simulink model "two_tank_simple"  (R2023b)
settings: Solver=ode45  StartTime=0.0  StopTime=199.9  RelTol=1e-3  EnableMultiTasking=on
values from neighbouring files (symbols this model uses):
  A1 = 0.0154    [INIT.m]
  A2 = 0.0154    [INIT.m]
  Cvb = 1.5938*1e-4    (= 0.00015938)    [INIT.m]
  Cvo = 1.59640*1e-4    (= 0.00015964)    [INIT.m]
  h1c = 0.5    [INIT.m]
  h1c_0 = 0    [INIT.m]
  h1max = 0.6    [INIT.m]
  h2c_0 = 0.03    [INIT.m]
  h2c_max = 0.11    [INIT.m]
  h2c_min = 0.09    [INIT.m]
  h2max = 0.6    [INIT.m]
  Ki = 5*1e-6    (= 5e-06)    [INIT.m]
  Kp = 1e-3    (= 0.001)    [INIT.m]
  Qf1 = 1e-4    (= 0.0001)    [INIT.m]    (also in extract_data.m = 5e-5*randn + 1e-4)
  Qf2 = 1e-4    (= 0.0001)    [INIT.m]    (also in extract_data.m = 5e-5*randn + 1e-4)
  Qpmax = 1e-2    (= 0.01)    [INIT.m]
  rate_noise_mQp = 1e-6    (= 1e-06)    [INIT.m]
  rate_noise_mUp = 1e-6    (= 1e-06)    [INIT.m]
  rate_noise_my1 = 1e-6    (= 1e-06)    [INIT.m]
  rate_noise_my2 = 1e-6    (= 1e-06)    [INIT.m]
  Te = 1    [INIT.m]
  yo = 0    [INIT.m]
(part 1 of 4)
settings Model: Creator=upcnet  LastModifiedBy=Plambeck
settings SolverCC: AlgebraicLoopSolver=TrustRegion
settings DataIOCC: LimitDataPoints=on  SaveFormat=Array  SignalLoggingSaveFormat=ModelDataLogs  ReturnWorkspaceOutputs=off  SignalLoggingName=sigsOut
settings OptimizationCC: BlockReduction=off  BooleanDataType=off  LifeSpan=inf
settings DebuggingCC: SaveWithParameterizedLinksMsg=none  UnderspecifiedInitializationDetection=Classic  MergeDetectMultiDrivingBlocksExec=none  SignalResolutionControl=TryResolveAllWithWarning  MultiTaskDSMMsg=warning  MultiTaskCondExecSysMsg=none  UnconnectedInputMsg=warning  UnconnectedOutputMsg=warning  UnconnectedLineMsg=warning  AllowSymbolicDim=off  SFUnexpectedBacktrackingDiag=warning  SFNoUnconditionalDefaultTransitionDiag=warning  SFExecutionAtInitializationDiag=none  ArithmeticOperatorsInVariantConditions=warning
settings HardwareCC: ProdBitPerPointer=32  ProdBitPerSizeT=32  ProdBitPerPtrDiffT=32  ProdLargestAtomicFloat=None  ProdIntDivRoundTo=Undefined  ProdEndianess=Unspecified  ProdWordSize=32  ProdHWDeviceType=32-bit Generic  TargetUnknown=on
settings ModelReferenceCC: EnableRefExpFcnMdlSchedulingChecks=on  PropagateSignalLabelsOutOfModel=off
settings SFSimCC: SimUseLocalCustomCode=off  CustomCodeUndefinedFunction=UseInterfaceOnly
settings RTWCC: RTWUseLocalCustomCode=off
settings CodeAppCC: StateflowObjectComments=on
settings GRTTargetCC: TargetLangStandard=C89/C90 (ANSI)  CombineOutputUpdateFcns=off  GRTInterface=on
settings ConfigComp: CovMetricSettings=dw  CovSaveCumulativeToWorkspaceVar=on  CovSaveSingleToWorkspaceVar=on  CovExternalEMLEnable=off

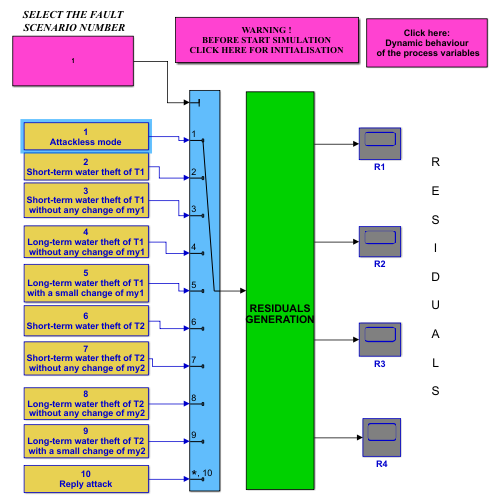
[thumbnail: Simulink's stored preview of the top-level diagram]
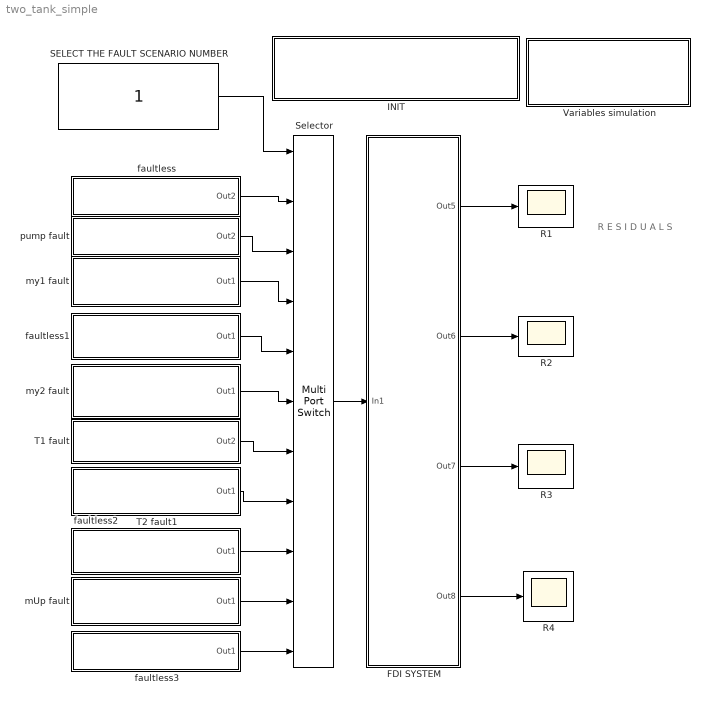
== system two_tank_simple ==
  note: R
      |
      | E
      |
      | S
      |
      | I
      |
      | D
      |
      | U
      |
      | A
      |
      | L
      |
      | S
  FDI SYSTEM : Subsystem
      mask Display: disp('\n\n\n\nRESIDUALS\nGENERATION')
  INIT : Subsystem
      settings: OpenFcn=INIT
      mask Display: disp('WARNING !\nBEFORE START SIMULATION\nCLICK HERE FOR INITIALISATION')
  R{1..4} (4 alike) : Scope
  SELECT THE FAULT SCENARIO NUMBER : Constant  Tag=cvcxv
  Selector : MultiPortSwitch  Inputs=10
  T1 fault : Subsystem
      mask Display: disp('6\nShort-term water theft of T2')
  T2 fault1 : Subsystem
      mask Display: disp('7\nShort-term water theft of T2\n without any change of my2')
  Variables simulation : Subsystem
      mask Display: disp('Click here:\nDynamic behaviour\n of the process variables')
  faultless : Subsystem
      mask Display: disp('1\nAttackless mode')
  faultless1 : Subsystem
      mask Display: disp('4\nLong-term water theft of T1\n without any change of my1')
  faultless2 : Subsystem
      mask Display: disp('8\nLong-term water theft of T2\n without any change of my2')
  faultless3 : Subsystem
      mask Display: disp('10\nReply attack')
  mUp fault : Subsystem
      mask Display: disp('9\nLong-term water theft of T2\n with a small change of my2')
  my1 fault : Subsystem
      mask Display: disp('3\nShort-term water theft of T1\n without any change of my1')
  my2 fault : Subsystem
      mask Display: disp('5\nLong-term water theft of T1\nwith a small change of my1')
  pump fault : Subsystem
      mask Display: disp('2\nShort-term water theft of T1')
  wires:
  faultless/1(Out2) -> Selector/2
  Selector/1 -> FDI SYSTEM/1(In1)
  pump fault/1(Out2) -> Selector/3
  SELECT THE FAULT SCENARIO NUMBER/1 -> Selector/1
  FDI SYSTEM/1(Out5) -> R1/1
  FDI SYSTEM/2(Out6) -> R2/1
  FDI SYSTEM/4(Out8) -> R4/1
  FDI SYSTEM/3(Out7) -> R3/1
  faultless3/1(Out1) -> Selector/11
  my1 fault/1(Out1) -> Selector/4
  my2 fault/1(Out1) -> Selector/6
  T1 fault/1(Out2) -> Selector/7
  T2 fault1/1(Out1) -> Selector/8
  faultless2/1(Out1) -> Selector/9
  faultless1/1(Out1) -> Selector/5
  mUp fault/1(Out1) -> Selector/10

== system two_tank_simple/FDI SYSTEM ==
  note: mQp
  note: mUb
  note: Uo
  note: my1
  note: my2
  note: h1c
  note: mUp
  note: R1
  note: R2
  note: R3
  note: R4
  note: Known
      | variables
  In1 : Inport
  Demux : Demux  Outputs=12
      settings: DisplayOption=none
  Digital Clock : DigitalClock  SampleTime=Te
  Mux : Mux
  Residuals generation : Subsystem
      mask Display: disp('Residuals\nGeneration\n using\nParity Space')
  To Workspace : ToWorkspace  VariableName=Resid  SampleTime=0.1
  To Workspace1 : ToWorkspace  VariableName=Monit  SampleTime=0.1
  To Workspace8 : ToWorkspace  VariableName=td  SampleTime=-1
  Out5 : Outport
  Out6 : Outport  Port=2
  Out7 : Outport  Port=3
  Out8 : Outport  Port=4
  tag scope: outputs=global
  wires:
  Demux/7 -> Residuals generation/7(In14)
  In1/1 -> To Workspace1/1, Demux/1, [outputs]
  Digital Clock/1 -> To Workspace8/1
  Residuals generation/1(Out1) -> Mux/1, Out5/1
  Residuals generation/2(Out2) -> Mux/2, Out6/1
  Residuals generation/3(Out3) -> Mux/3, Out7/1
  Residuals generation/4(Out4) -> Mux/4, Out8/1
  Demux/6 -> Residuals generation/6(In8)
  Demux/5 -> Residuals generation/5(In13)
  Demux/4 -> Residuals generation/4(In12)
  Demux/3 -> Residuals generation/3(In11)
  Demux/2 -> Residuals generation/2(In10)
  Demux/1 -> Residuals generation/1(mQp)
  Mux/1 -> To Workspace/1

== system two_tank_simple/INIT ==

== system two_tank_simple/T1 fault ==
  note: mQp
  note: mUb
  note: Uo
  note: my1
  note: my2
  note: h1c
  note: mUp
  note: y2
  note: vol2
  note: y1
  note: vol1
  note: mQ0
  FAULTLESS FAULT : Subsystem
      mask Display: disp('P\nR\nO\nC\nE\nS\nS')
  Mux1 : Mux  Inputs=12
  Out2 : Outport
  wires:
  FAULTLESS FAULT/1(mQp) -> Mux1/1
  FAULTLESS FAULT/2(mUb) -> Mux1/2
  FAULTLESS FAULT/3("Uo ") -> Mux1/3
  FAULTLESS FAULT/4(my1) -> Mux1/4
  FAULTLESS FAULT/6(h1c) -> Mux1/6
  FAULTLESS FAULT/7(mUp) -> Mux1/7
  FAULTLESS FAULT/5(my2) -> Mux1/5
  Mux1/1 -> Out2/1
  FAULTLESS FAULT/8(mq0) -> Mux1/8
  FAULTLESS FAULT/9(y1) -> Mux1/9
  FAULTLESS FAULT/10(vol1) -> Mux1/10
  FAULTLESS FAULT/11(y2) -> Mux1/11
  FAULTLESS FAULT/12(vol2) -> Mux1/12

== system two_tank_simple/T2 fault1 ==
  note: mQp
  note: mUb
  note: Uo
  note: my1
  note: my2
  note: h1c
  note: mUp
  note: y2
  note: vol2
  note: y1
  note: vol1
  note: mQ0
  FAULTLESS FAULT : Subsystem
      mask Display: disp('P\nR\nO\nC\nE\nS\nS')
  Mux : Mux  Inputs=12
  Out1 : Outport
  wires:
  FAULTLESS FAULT/1(mQp) -> Mux/1
  FAULTLESS FAULT/2(mUb) -> Mux/2
  FAULTLESS FAULT/3("Uo ") -> Mux/3
  FAULTLESS FAULT/4(my1) -> Mux/4
  FAULTLESS FAULT/6(h1c) -> Mux/6
  FAULTLESS FAULT/7(mUp) -> Mux/7
  FAULTLESS FAULT/5(my2) -> Mux/5
  Mux/1 -> Out1/1
  FAULTLESS FAULT/8(mQ0) -> Mux/8
  FAULTLESS FAULT/9(vol1) -> Mux/9
  FAULTLESS FAULT/10(y1) -> Mux/10
  FAULTLESS FAULT/11(y2) -> Mux/11
  FAULTLESS FAULT/12(vol2) -> Mux/12

== system two_tank_simple/Variables simulation ==
  Demux : Demux  Outputs=12
      settings: DisplayOption=none
  To Workspace : ToWorkspace  VariableName=output  SampleTime=0.1
  Uo : Scope
  h1c : Scope
  mQ0 : Scope
  mQp : Scope
  mUb : Scope
  mUp : Scope
  my1 : Scope
  my2 : Scope
  vol1 : Scope
  vol2 : Scope
  y1 : Scope
  y2 : Scope
  wires:
  [outputs] -> To Workspace/1, Demux/1
  Demux/1 -> mQp/1
  Demux/2 -> mUb/1
  Demux/3 -> Uo/1
  Demux/4 -> my1/1
  Demux/5 -> my2/1
  Demux/6 -> h1c/1
  Demux/7 -> mUp/1
  Demux/12 -> vol2/1
  Demux/11 -> y2/1
  Demux/10 -> vol1/1
  Demux/9 -> y1/1
  Demux/8 -> mQ0/1

== system two_tank_simple/faultless ==
  note: mQp
  note: mUb
  note: Uo
  note: my1
  note: my2
  note: h1c
  note: mUp
  note: y2
  note: vol2
  note: y1
  note: vol1
  note: mQ0
  FAULTLESS FAULT : Subsystem
      mask Display: disp('P\nR\nO\nC\nE\nS\nS')
  Mux1 : Mux  Inputs=12
  Out2 : Outport
  wires:
  FAULTLESS FAULT/1(mQp) -> Mux1/1
  FAULTLESS FAULT/2(mUb) -> Mux1/2
  FAULTLESS FAULT/3("Uo ") -> Mux1/3
  FAULTLESS FAULT/4(my1) -> Mux1/4
  FAULTLESS FAULT/6(h1c) -> Mux1/6
  FAULTLESS FAULT/7(mUp) -> Mux1/7
  FAULTLESS FAULT/5(my2) -> Mux1/5
  Mux1/1 -> Out2/1
  FAULTLESS FAULT/8(mq0) -> Mux1/8
  FAULTLESS FAULT/9(y1) -> Mux1/9
  FAULTLESS FAULT/10(vol1) -> Mux1/10
  FAULTLESS FAULT/11(y2) -> Mux1/11
  FAULTLESS FAULT/12(vol2) -> Mux1/12

== system two_tank_simple/faultless1 ==
  note: mQp
  note: mUb
  note: Uo
  note: my1
  note: my2
  note: h1c
  note: mUp
  note: mq0
  note: y1
  note: vol1
  note: y2
  note: vol2
  FAULTLESS FAULT : Subsystem
      mask Display: disp('P\nR\nO\nC\nE\nS\nS')
  Mux : Mux  Inputs=12
  Out1 : Outport
  wires:
  FAULTLESS FAULT/1(mQp) -> Mux/1
  FAULTLESS FAULT/2(mUb) -> Mux/2
  FAULTLESS FAULT/3("Uo ") -> Mux/3
  FAULTLESS FAULT/4(my1) -> Mux/4
  FAULTLESS FAULT/6(h1c) -> Mux/6
  FAULTLESS FAULT/7(mUp) -> Mux/7
  FAULTLESS FAULT/5(my2) -> Mux/5
  Mux/1 -> Out1/1
  FAULTLESS FAULT/8(mq0) -> Mux/8
  FAULTLESS FAULT/9(y1) -> Mux/9
  FAULTLESS FAULT/10(vol1) -> Mux/10
  FAULTLESS FAULT/11(y2) -> Mux/11
  FAULTLESS FAULT/12(vol2) -> Mux/12

== system two_tank_simple/faultless2 ==
  note: mQp
  note: mUb
  note: Uo
  note: my1
  note: my2
  note: h1c
  note: mUp
  note: y2
  note: vol2
  note: y1
  note: vol1
  note: mQ0
  FAULTLESS FAULT : Subsystem
      mask Display: disp('P\nR\nO\nC\nE\nS\nS')
  Mux : Mux  Inputs=12
  Out1 : Outport
  wires:
  FAULTLESS FAULT/1(mQp) -> Mux/1
  FAULTLESS FAULT/2(mUb) -> Mux/2
  FAULTLESS FAULT/3("Uo ") -> Mux/3
  FAULTLESS FAULT/4(my1) -> Mux/4
  FAULTLESS FAULT/6(h1c) -> Mux/6
  FAULTLESS FAULT/7(mUp) -> Mux/7
  FAULTLESS FAULT/5(my2) -> Mux/5
  Mux/1 -> Out1/1
  FAULTLESS FAULT/8(mQ0) -> Mux/8
  FAULTLESS FAULT/9(y1) -> Mux/9
  FAULTLESS FAULT/10(vol1) -> Mux/10
  FAULTLESS FAULT/11(y2) -> Mux/11
  FAULTLESS FAULT/12(vol2) -> Mux/12

== system two_tank_simple/faultless3 ==
  note: mQp
  note: mUb
  note: Uo
  note: my1
  note: my2
  note: h1c
  note: mUp
  note: y2
  note: vol2
  note: y1
  note: vol1
  note: mQ0
  FAULTLESS FAULT : Subsystem
      mask Display: disp('P\nR\nO\nC\nE\nS\nS')
  Mux : Mux  Inputs=12
  Out1 : Outport
  wires:
  FAULTLESS FAULT/1(mQp) -> Mux/1
  FAULTLESS FAULT/2(mUb) -> Mux/2
  FAULTLESS FAULT/3("Uo ") -> Mux/3
  FAULTLESS FAULT/4(my1) -> Mux/4
  FAULTLESS FAULT/6(h1c) -> Mux/6
  FAULTLESS FAULT/7(mUp) -> Mux/7
  FAULTLESS FAULT/5(my2) -> Mux/5
  Mux/1 -> Out1/1
  FAULTLESS FAULT/8(mQ0) -> Mux/8
  FAULTLESS FAULT/9(y1) -> Mux/9
  FAULTLESS FAULT/10(vol1) -> Mux/10
  FAULTLESS FAULT/11(y2) -> Mux/11
  FAULTLESS FAULT/12(vol2) -> Mux/12

== system two_tank_simple/mUp fault ==
  note: mQp
  note: mUb
  note: Uo
  note: my1
  note: my2
  note: h1c
  note: mUp
  note: y2
  note: vol2
  note: y1
  note: vol1
  note: mQ0
  FAULTLESS FAULT : Subsystem
      mask Display: disp('P\nR\nO\nC\nE\nS\nS')
  Mux : Mux  Inputs=12
  Out1 : Outport
  wires:
  FAULTLESS FAULT/1(mQp) -> Mux/1
  FAULTLESS FAULT/2(mUb) -> Mux/2
  FAULTLESS FAULT/3("Uo ") -> Mux/3
  FAULTLESS FAULT/4(my1) -> Mux/4
  FAULTLESS FAULT/6(h1c) -> Mux/6
  FAULTLESS FAULT/7(mUp) -> Mux/7
  FAULTLESS FAULT/5(my2) -> Mux/5
  Mux/1 -> Out1/1
  FAULTLESS FAULT/8(mQ0) -> Mux/8
  FAULTLESS FAULT/9(vol1) -> Mux/9
  FAULTLESS FAULT/10(y1) -> Mux/10
  FAULTLESS FAULT/11(y2) -> Mux/11
  FAULTLESS FAULT/12(vol2) -> Mux/12

== system two_tank_simple/my1 fault ==
  note: mQp
  note: mUb
  note: Uo
  note: my1
  note: my2
  note: h1c
  note: mUp
  note: y2
  note: vol2
  note: y1
  note: vol1
  note: mQ0
  FAULTLESS FAULT : Subsystem
      mask Display: disp('P\nR\nO\nC\nE\nS\nS')
  Mux : Mux  Inputs=12
  Out1 : Outport
  wires:
  FAULTLESS FAULT/1(mQp) -> Mux/1
  FAULTLESS FAULT/2(mUb) -> Mux/2
  FAULTLESS FAULT/3("Uo ") -> Mux/3
  FAULTLESS FAULT/4(my1) -> Mux/4
  FAULTLESS FAULT/6(h1c) -> Mux/6
  FAULTLESS FAULT/7(mUp) -> Mux/7
  FAULTLESS FAULT/5(my2) -> Mux/5
  Mux/1 -> Out1/1
  FAULTLESS FAULT/8(mq0) -> Mux/8
  FAULTLESS FAULT/9(y1) -> Mux/9
  FAULTLESS FAULT/10(vol1) -> Mux/10
  FAULTLESS FAULT/11(y2) -> Mux/11
  FAULTLESS FAULT/12(vol2) -> Mux/12

== system two_tank_simple/my2 fault ==
  note: mQp
  note: mUb
  note: Uo
  note: my1
  note: my2
  note: h1c
  note: mUp
  note: mq0
  note: y1
  note: vol1
  note: y2
  note: vol2
  FAULTLESS FAULT : Subsystem
      mask Display: disp('P\nR\nO\nC\nE\nS\nS')
  Mux : Mux  Inputs=12
  Out1 : Outport
  wires:
  FAULTLESS FAULT/1(mQp) -> Mux/1
  FAULTLESS FAULT/2(mUb) -> Mux/2
  FAULTLESS FAULT/3("Uo ") -> Mux/3
  FAULTLESS FAULT/4(my1) -> Mux/4
  FAULTLESS FAULT/6(h1c) -> Mux/6
  FAULTLESS FAULT/7(mUp) -> Mux/7
  FAULTLESS FAULT/5(my2) -> Mux/5
  Mux/1 -> Out1/1
  FAULTLESS FAULT/8(mq0) -> Mux/8
  FAULTLESS FAULT/9(y1) -> Mux/9
  FAULTLESS FAULT/10(vol1) -> Mux/10
  FAULTLESS FAULT/11(y2) -> Mux/11
  FAULTLESS FAULT/12(vol2) -> Mux/12

== system two_tank_simple/pump fault ==
  note: mQp
  note: mUb
  note: Uo
  note: my1
  note: my2
  note: h1c
  note: mUp
  note: y2
  note: vol2
  note: y1
  note: vol1
  note: mQ0
  FAULTLESS FAULT : Subsystem
      mask Display: disp('P\nR\nO\nC\nE\nS\nS')
  Mux1 : Mux  Inputs=12
  Out2 : Outport
  wires:
  FAULTLESS FAULT/1(mQp) -> Mux1/1
  FAULTLESS FAULT/2(mUb) -> Mux1/2
  FAULTLESS FAULT/3("Uo ") -> Mux1/3
  FAULTLESS FAULT/4(my1) -> Mux1/4
  FAULTLESS FAULT/6(h1c) -> Mux1/6
  FAULTLESS FAULT/7(mUp) -> Mux1/7
  FAULTLESS FAULT/5(my2) -> Mux1/5
  Mux1/1 -> Out2/1
  FAULTLESS FAULT/9(y1) -> Mux1/9
  FAULTLESS FAULT/10(vol1) -> Mux1/10
  FAULTLESS FAULT/11(y2) -> Mux1/11
  FAULTLESS FAULT/12(vol2) -> Mux1/12
  FAULTLESS FAULT/8(mq0) -> Mux1/8

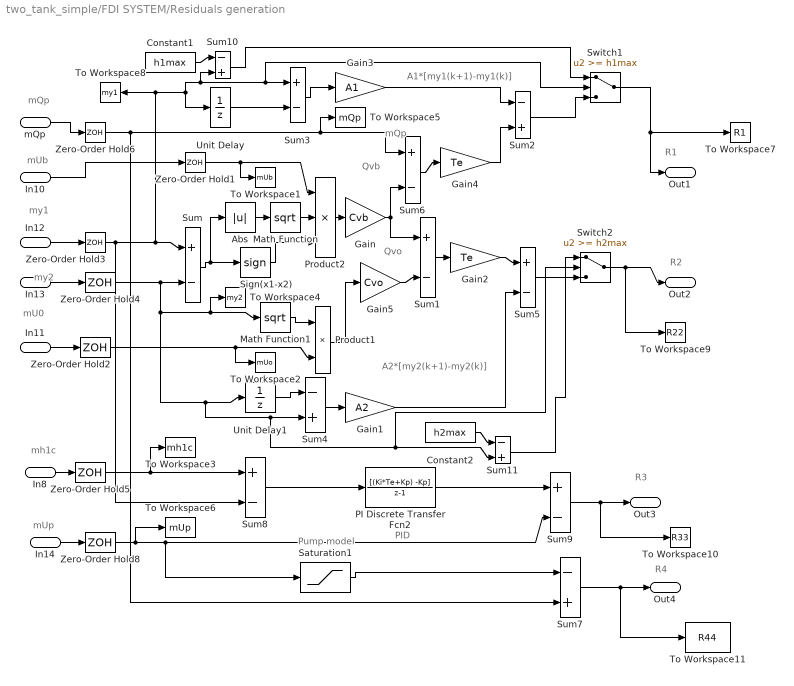
== system two_tank_simple/FDI SYSTEM/Residuals generation ==
  note: my1
  note: my2
  note: mUb
  note: mU0
  note: mUp
  note: A2*[my2(k+1)-my2(k)]
  note: mQp
  note: Qvb
  note: Qvo
  note: A1*[my1(k+1)-my1(k)]
  note: mh1c
  note: R1
  note: R2
  note: R3
  note: R4
  note: PID
  note: Pump model
  note: mQp
  mQp : Inport
  In10 : Inport  Port=2
  In11 : Inport  Port=3
  In12 : Inport  Port=4
  In13 : Inport  Port=5
  In8 : Inport  Port=6
  In14 : Inport  Port=7
  Abs : Abs
  Constant1 : Constant  Value=h1max
  Constant2 : Constant  Value=h2max
  Gain : Gain  Gain=Cvb  SaturateOnIntegerOverflow=on  OutDataTypeStr=Inherit: Same as input  ParamDataTypeStr=Inherit: Same as input
  Gain1 : Gain  Gain=A2  SaturateOnIntegerOverflow=on  OutDataTypeStr=Inherit: Same as input  ParamDataTypeStr=Inherit: Same as input
  Gain2 : Gain  Gain=Te  SaturateOnIntegerOverflow=on  OutDataTypeStr=Inherit: Same as input  ParamDataTypeStr=Inherit: Same as input
  Gain3 : Gain  Gain=A1  SaturateOnIntegerOverflow=on  OutDataTypeStr=Inherit: Same as input  ParamDataTypeStr=Inherit: Same as input
  Gain4 : Gain  Gain=Te  SaturateOnIntegerOverflow=on  OutDataTypeStr=Inherit: Same as input  ParamDataTypeStr=Inherit: Same as input
  Gain5 : Gain  Gain=Cvo  SaturateOnIntegerOverflow=on  OutDataTypeStr=Inherit: Same as input  ParamDataTypeStr=Inherit: Same as input
  Math Function : Math  Operator=sqrt  SignedPower=on
  Math Function1 : Math  Operator=sqrt  SignedPower=on
  PI Discrete Transfer Fcn2 : DiscreteTransferFcn  Numerator=[(Ki*Te+Kp) -Kp]  Denominator=[1 -1]  SampleTime=Te
  Product1 : Product  InputSameDT=on  SaturateOnIntegerOverflow=on  OutDataTypeStr=Inherit: Same as first input
  Product2 : Product  Inputs=3  InputSameDT=on  SaturateOnIntegerOverflow=on  OutDataTypeStr=Inherit: Same as first input
  Saturation1 : Saturate  UpperLimit=Qpmax  LowerLimit=0
  Sign(x1-x2) : Signum
  Sum{,1,3,5..6,8..9} (7 alike) : Sum  Inputs=+-  InputSameDT=on  SaturateOnIntegerOverflow=on  OutDataTypeStr=Inherit: Same as first input
  Sum{2,4,7,10..11} (5 alike) : Sum  Inputs=-+  InputSameDT=on  SaturateOnIntegerOverflow=on  OutDataTypeStr=Inherit: Same as first input
  Switch1 : Switch  Threshold=h1max
  Switch2 : Switch  Threshold=h2max
  To Workspace1 : ToWorkspace  VariableName=mUb  SampleTime=-1
  To Workspace10 : ToWorkspace  VariableName=R33  SampleTime=-1
  To Workspace11 : ToWorkspace  VariableName=R44  SampleTime=-1
  To Workspace2 : ToWorkspace  VariableName=mUo  SampleTime=-1
  To Workspace3 : ToWorkspace  VariableName=mh1c  SampleTime=-1
  To Workspace4 : ToWorkspace  VariableName=my2  SampleTime=-1
  To Workspace5 : ToWorkspace  VariableName=mQp  SampleTime=-1
  To Workspace6 : ToWorkspace  VariableName=mUp  SampleTime=-1
  To Workspace7 : ToWorkspace  VariableName=R1  SampleTime=-1
  To Workspace8 : ToWorkspace  VariableName=my1  SampleTime=-1
  To Workspace9 : ToWorkspace  VariableName=R22  SampleTime=-1
  Unit Delay : UnitDelay  SampleTime=Te  HasFrameUpgradeWarning=on
  Unit Delay1 : UnitDelay  SampleTime=Te  HasFrameUpgradeWarning=on
  Zero-Order Hold{1..6,8} (7 alike) : ZeroOrderHold  SampleTime=Te
  Out1 : Outport  InitialOutput=0
  Out2 : Outport  Port=2  InitialOutput=0
  Out3 : Outport  Port=3  InitialOutput=0
  Out4 : Outport  Port=4  InitialOutput=0
  wires:
  Unit Delay/1 -> Sum3/2
  Sum6/1 -> Gain4/1
  Gain1/1 -> Sum5/2
  Gain2/1 -> Sum5/1
  Sum1/1 -> Gain2/1
  Sum4/1 -> Gain1/1
  Unit Delay1/1 -> Sum4/1
  Sum3/1 -> Gain3/1
  In13/1 -> Zero-Order Hold4/1
  Zero-Order Hold4/1 -> Unit Delay1/1, Sum4/2, Sum11/2, Switch2/2, To Workspace4/1, Math Function1/1, Sum/2
  In12/1 -> Zero-Order Hold3/1
  Zero-Order Hold3/1 -> Sum/1, Unit Delay/1, Sum3/1, Switch1/2, Sum10/2, To Workspace8/1, Sum8/2
  In11/1 -> Zero-Order Hold2/1
  In10/1 -> Zero-Order Hold1/1
  Zero-Order Hold1/1 -> Product2/1, To Workspace1/1
  Sum/1 -> Sign(x1-x2)/1, Abs/1
  Sign(x1-x2)/1 -> Product2/3
  Product2/1 -> Gain/1
  Gain/1 -> Sum6/2, Sum1/1
  Math Function/1 -> Product2/2
  Abs/1 -> Math Function/1
  Zero-Order Hold2/1 -> Product1/2, To Workspace2/1
  Product1/1 -> Gain5/1
  Gain5/1 -> Sum1/2
  Saturation1/1 -> Sum7/1
  Zero-Order Hold8/1 -> Sum9/2, Saturation1/1, To Workspace6/1
  Sum9/1 -> Out3/1, To Workspace10/1
  Sum7/1 -> Out4/1, To Workspace11/1
  Zero-Order Hold6/1 -> Sum6/1, To Workspace5/1, Sum7/2
  mQp/1 -> Zero-Order Hold6/1
  In8/1 -> Zero-Order Hold5/1
  Zero-Order Hold5/1 -> Sum8/1, To Workspace3/1
  In14/1 -> Zero-Order Hold8/1
  PI Discrete Transfer Fcn2/1 -> Sum9/1
  Sum8/1 -> PI Discrete Transfer Fcn2/1
  Gain3/1 -> Sum2/1
  Gain4/1 -> Sum2/2
  Sum2/1 -> Switch1/3
  Constant1/1 -> Sum10/1
  Sum10/1 -> Switch1/1
  Switch1/1 -> Out1/1, To Workspace7/1
  Sum5/1 -> Switch2/3
  Sum11/1 -> Switch2/1
  Constant2/1 -> Sum11/1
  Switch2/1 -> Out2/1, To Workspace9/1
  Math Function1/1 -> Product1/1

== system two_tank_simple/T1 fault/FAULTLESS FAULT ==
  note: y2
  note: y1
  note: Ub
  note: Up
  note: Qvo
      | To users
  note: Qp
  note: Qvb
  Constant : Constant  Value=yo
  Subsystem1 : Subsystem
      mask Display: disp('TANK 1')
  Subsystem10 : Subsystem
      mask Display: disp('Sensor\n y2')
  Subsystem11 : Subsystem
      mask Display: disp('Controller 1')
  Subsystem12 : Subsystem
      mask Display: disp('Sensor\n Ub')
  Subsystem13 : Subsystem
      mask Display: disp('Sensor\n Up')
  Subsystem14 : Subsystem
      mask Display: disp('Sensor\n Qp')
  Subsystem2 : Subsystem
      mask Display: disp('Valve B')
  Subsystem3 : Subsystem
      mask Display: disp('Valve O')
  Subsystem4 : Subsystem
      mask Display: disp('Controller2')
  Subsystem6 : Subsystem
      mask Display: disp('Pump')
  Subsystem7 : Subsystem
      mask Display: disp('Sensor\n y1')
  Subsystem8 : Subsystem
      mask Display: disp('TANK 2')
  Subsystem9 : Subsystem
      mask Display: disp('OPERATOR\nSET')
  mQp : Outport
  mUb : Outport  Port=2
  "Uo " : Outport  Port=3
  my1 : Outport  Port=4
  my2 : Outport  Port=5
  h1c : Outport  Port=6
  mUp : Outport  Port=7
  mq0 : Outport  Port=8
  y1 : Outport  Port=9
  vol1 : Outport  Port=10
  y2 : Outport  Port=11
  vol2 : Outport  Port=12
  wires:
  Subsystem1/1(y1) -> Subsystem2/2(y1), Subsystem7/1(In1)
  Subsystem12/1(mUb) -> mUb/1
  Subsystem3/1(Qv0) -> mq0/1, Subsystem8/1(Qvo)
  Constant/1 -> Subsystem3/3(y0)
  Subsystem13/1(mUp) -> mUp/1
  Subsystem8/1(y2) -> Subsystem3/2(y2), Subsystem2/3(y2), Subsystem10/1(y2)
  Subsystem2/1(QVb) -> Subsystem8/2(Qvb), Subsystem1/2(Qvb)
  Subsystem11/1(mUp) -> Subsystem13/1(Up), Subsystem6/1(Up)
  Subsystem9/1(Out3) -> Subsystem11/1(h1c), h1c/1
  Subsystem9/2(Out1) -> "Uo "/1, Subsystem3/1(U0)
  Subsystem7/1(Out5) -> Subsystem11/2(my1), my1/1
  Subsystem14/1(mQp) -> mQp/1
  Subsystem4/1(Out5) -> Subsystem12/1(Ub), Subsystem2/1(Ub)
  Subsystem10/1(my2) -> my2/1, Subsystem4/1(In2)
  Subsystem6/1(mUp) -> Subsystem1/1(Qp), Subsystem14/1(Qp)
  Subsystem10/3(vol2) -> vol2/1
  Subsystem10/2(yy2) -> y2/1
  Subsystem7/2(Out1) -> y1/1
  Subsystem7/3(Out2) -> vol1/1

== system two_tank_simple/T2 fault1/FAULTLESS FAULT ==
  note: y2
  note: y1
  note: Ub
  note: Up
  note: Qvo
      | To users
  note: Qp
  note: Qvb
  Constant : Constant  Value=yo
  Subsystem1 : Subsystem
      mask Display: disp('TANK 1')
  Subsystem10 : Subsystem
      mask Display: disp('Sensor\n y2')
  Subsystem11 : Subsystem
      mask Display: disp('Controller 1')
  Subsystem12 : Subsystem
      mask Display: disp('Sensor\n Ub')
  Subsystem13 : Subsystem
      mask Display: disp('Sensor\n Up')
  Subsystem14 : Subsystem
      mask Display: disp('Sensor\n Qp')
  Subsystem2 : Subsystem
      mask Display: disp('Valve B')
  Subsystem3 : Subsystem
      mask Display: disp('Valve O')
  Subsystem4 : Subsystem
      mask Display: disp('Controller2')
  Subsystem6 : Subsystem
      mask Display: disp('Pump')
  Subsystem7 : Subsystem
      mask Display: disp('Sensor\n y1')
  Subsystem8 : Subsystem
      mask Display: disp('TANK 2')
  Subsystem9 : Subsystem
      mask Display: disp('OPERATOR\nSET')
  mQp : Outport
  mUb : Outport  Port=2
  "Uo " : Outport  Port=3
  my1 : Outport  Port=4
  my2 : Outport  Port=5
  h1c : Outport  Port=6
  mUp : Outport  Port=7
  mQ0 : Outport  Port=8
  vol1 : Outport  Port=9
  y1 : Outport  Port=10
  y2 : Outport  Port=11
  vol2 : Outport  Port=12
  wires:
  Subsystem1/1(y1) -> Subsystem2/2(y1), Subsystem7/1(In1)
  Subsystem12/1(mUb) -> mUb/1
  Subsystem3/1(Qv0) -> mQ0/1, Subsystem8/1(Qvo)
  Constant/1 -> Subsystem3/3(y0)
  Subsystem13/1(mUp) -> mUp/1
  Subsystem8/1(y2) -> Subsystem3/2(y2), Subsystem2/3(y2), Subsystem10/1(y2)
  Subsystem2/1(QVb) -> Subsystem8/2(Qvb), Subsystem1/2(Qvb)
  Subsystem11/1(mUp) -> Subsystem13/1(Up), Subsystem6/1(Up)
  Subsystem9/1(Out3) -> Subsystem11/1(h1c), h1c/1
  Subsystem9/2(Out1) -> "Uo "/1, Subsystem3/1(U0)
  Subsystem7/1(Out5) -> Subsystem11/2(my1), my1/1
  Subsystem14/1(mQp) -> mQp/1
  Subsystem4/1(Out5) -> Subsystem12/1(Ub), Subsystem2/1(Ub)
  Subsystem10/1(my2) -> my2/1, Subsystem4/1(In2)
  Subsystem6/1(mUp) -> Subsystem1/1(Qp), Subsystem14/1(Qp)
  Subsystem7/3(Out2) -> y1/1
  Subsystem7/2(Out1) -> vol1/1
  Subsystem10/2(yy2) -> y2/1
  Subsystem10/3(vol2) -> vol2/1

== system two_tank_simple/faultless/FAULTLESS FAULT ==
  note: y2
  note: y1
  note: Ub
  note: Up
  note: Qvo
      | To users
  note: Qp
  note: Qvb
  Constant : Constant  Value=yo
  Subsystem1 : Subsystem
      mask Display: disp('TANK 1')
  Subsystem10 : Subsystem
      mask Display: disp('Sensor\n y2')
  Subsystem11 : Subsystem
      mask Display: disp('Controller 1')
  Subsystem12 : Subsystem
      mask Display: disp('Sensor\n Ub')
  Subsystem13 : Subsystem
      mask Display: disp('Sensor\n Up')
  Subsystem14 : Subsystem
      mask Display: disp('Sensor\n Qp')
  Subsystem2 : Subsystem
      mask Display: disp('Valve B')
  Subsystem3 : Subsystem
      mask Display: disp('Valve O')
  Subsystem4 : Subsystem
      mask Display: disp('Controller2')
  Subsystem6 : Subsystem
      mask Display: disp('Pump')
  Subsystem7 : Subsystem
      mask Display: disp('Sensor\n y1')
  Subsystem8 : Subsystem
      mask Display: disp('TANK 2')
  Subsystem9 : Subsystem
      mask Display: disp('OPERATOR\nSET')
  mQp : Outport
  mUb : Outport  Port=2
  "Uo " : Outport  Port=3
  my1 : Outport  Port=4
  my2 : Outport  Port=5
  h1c : Outport  Port=6
  mUp : Outport  Port=7
  mq0 : Outport  Port=8
  y1 : Outport  Port=9
  vol1 : Outport  Port=10
  y2 : Outport  Port=11
  vol2 : Outport  Port=12
  wires:
  Subsystem1/1(y1) -> Subsystem2/2(y1), Subsystem7/1(In1)
  Subsystem12/1(mUb) -> mUb/1
  Subsystem3/1(Qv0) -> mq0/1, Subsystem8/1(Qvo)
  Constant/1 -> Subsystem3/3(y0)
  Subsystem13/1(mUp) -> mUp/1
  Subsystem8/1(y2) -> Subsystem3/2(y2), Subsystem2/3(y2), Subsystem10/1(y2)
  Subsystem2/1(QVb) -> Subsystem8/2(Qvb), Subsystem1/2(Qvb)
  Subsystem11/1(mUp) -> Subsystem13/1(Up), Subsystem6/1(Up)
  Subsystem9/1(Out3) -> Subsystem11/1(h1c), h1c/1
  Subsystem9/2(Out1) -> "Uo "/1, Subsystem3/1(U0)
  Subsystem7/1(Out5) -> Subsystem11/2(my1), my1/1
  Subsystem14/1(mQp) -> mQp/1
  Subsystem4/1(Out5) -> Subsystem12/1(Ub), Subsystem2/1(Ub)
  Subsystem10/1(my2) -> my2/1, Subsystem4/1(In2)
  Subsystem6/1(mUp) -> Subsystem1/1(Qp), Subsystem14/1(Qp)
  Subsystem10/3(vol2) -> vol2/1
  Subsystem10/2(yy2) -> y2/1
  Subsystem7/3(Out2) -> vol1/1
  Subsystem7/2(Out1) -> y1/1

== system two_tank_simple/faultless1/FAULTLESS FAULT ==
  note: y2
  note: y1
  note: Ub
  note: Up
  note: Qvo
      | To users
  note: Qp
  note: Qvb
  Constant : Constant  Value=yo
  Subsystem1 : Subsystem
      mask Display: disp('TANK 1')
  Subsystem10 : Subsystem
      mask Display: disp('Sensor\n y2')
  Subsystem11 : Subsystem
      mask Display: disp('Controller 1')
  Subsystem12 : Subsystem
      mask Display: disp('Sensor\n Ub')
  Subsystem13 : Subsystem
      mask Display: disp('Sensor\n Up')
  Subsystem14 : Subsystem
      mask Display: disp('Sensor\n Qp')
  Subsystem2 : Subsystem
      mask Display: disp('Valve B')
  Subsystem3 : Subsystem
      mask Display: disp('Valve O')
  Subsystem4 : Subsystem
      mask Display: disp('Controller2')
  Subsystem6 : Subsystem
      mask Display: disp('Pump')
  Subsystem7 : Subsystem
      mask Display: disp('Sensor\n y1')
  Subsystem8 : Subsystem
      mask Display: disp('TANK 2')
  Subsystem9 : Subsystem
      mask Display: disp('OPERATOR\nSET')
  mQp : Outport
  mUb : Outport  Port=2
  "Uo " : Outport  Port=3
  my1 : Outport  Port=4
  my2 : Outport  Port=5
  h1c : Outport  Port=6
  mUp : Outport  Port=7
  mq0 : Outport  Port=8
  y1 : Outport  Port=9
  vol1 : Outport  Port=10
  y2 : Outport  Port=11
  vol2 : Outport  Port=12
  wires:
  Subsystem1/1(y1) -> Subsystem2/2(y1), Subsystem7/1(In1)
  Subsystem12/1(mUb) -> mUb/1
  Subsystem3/1(Qv0) -> Subsystem8/1(Qvo), mq0/1
  Constant/1 -> Subsystem3/3(y0)
  Subsystem13/1(mUp) -> mUp/1
  Subsystem8/1(y2) -> Subsystem3/2(y2), Subsystem2/3(y2), Subsystem10/1(y2)
  Subsystem2/1(QVb) -> Subsystem8/2(Qvb), Subsystem1/2(Qvb)
  Subsystem11/1(mUp) -> Subsystem13/1(Up), Subsystem6/1(Up)
  Subsystem9/1(Out3) -> Subsystem11/1(h1c), h1c/1
  Subsystem9/2(Out1) -> "Uo "/1, Subsystem3/1(U0)
  Subsystem7/1(Out5) -> Subsystem11/2(my1), my1/1
  Subsystem14/1(mQp) -> mQp/1
  Subsystem4/1(Out5) -> Subsystem12/1(Ub), Subsystem2/1(Ub)
  Subsystem10/1(my2) -> my2/1, Subsystem4/1(In2)
  Subsystem6/1(mUp) -> Subsystem1/1(Qp), Subsystem14/1(Qp)
  Subsystem7/2(Out1) -> y1/1
  Subsystem7/3(Out2) -> vol1/1
  Subsystem10/2(yy2) -> y2/1
  Subsystem10/3(vol2) -> vol2/1

== system two_tank_simple/faultless2/FAULTLESS FAULT ==
  note: y2
  note: y1
  note: Ub
  note: Up
  note: Qvo
      | To users
  note: Qp
  note: Qvb
  Constant : Constant  Value=yo
  Subsystem1 : Subsystem
      mask Display: disp('TANK 1')
  Subsystem10 : Subsystem
      mask Display: disp('Sensor\n y2')
  Subsystem11 : Subsystem
      mask Display: disp('Controller 1')
  Subsystem12 : Subsystem
      mask Display: disp('Sensor\n Ub')
  Subsystem13 : Subsystem
      mask Display: disp('Sensor\n Up')
  Subsystem14 : Subsystem
      mask Display: disp('Sensor\n Qp')
  Subsystem2 : Subsystem
      mask Display: disp('Valve B')
  Subsystem3 : Subsystem
      mask Display: disp('Valve O')
  Subsystem4 : Subsystem
      mask Display: disp('Controller2')
  Subsystem6 : Subsystem
      mask Display: disp('Pump')
  Subsystem7 : Subsystem
      mask Display: disp('Sensor\n y1')
  Subsystem8 : Subsystem
      mask Display: disp('TANK 2')
  Subsystem9 : Subsystem
      mask Display: disp('OPERATOR\nSET')
  mQp : Outport
  mUb : Outport  Port=2
  "Uo " : Outport  Port=3
  my1 : Outport  Port=4
  my2 : Outport  Port=5
  h1c : Outport  Port=6
  mUp : Outport  Port=7
  mQ0 : Outport  Port=8
  y1 : Outport  Port=9
  vol1 : Outport  Port=10
  y2 : Outport  Port=11
  vol2 : Outport  Port=12
  wires:
  Subsystem1/1(y1) -> Subsystem2/2(y1), Subsystem7/1(In1)
  Subsystem12/1(mUb) -> mUb/1
  Subsystem3/1(Qv0) -> mQ0/1, Subsystem8/1(Qvo)
  Constant/1 -> Subsystem3/3(y0)
  Subsystem13/1(mUp) -> mUp/1
  Subsystem8/1(y2) -> Subsystem3/2(y2), Subsystem2/3(y2), Subsystem10/1(y2)
  Subsystem2/1(QVb) -> Subsystem8/2(Qvb), Subsystem1/2(Qvb)
  Subsystem11/1(mUp) -> Subsystem13/1(Up), Subsystem6/1(Up)
  Subsystem9/1(Out3) -> Subsystem11/1(h1c), h1c/1
  Subsystem9/2(Out1) -> "Uo "/1, Subsystem3/1(U0)
  Subsystem7/1(Out5) -> Subsystem11/2(my1), my1/1
  Subsystem14/1(mQp) -> mQp/1
  Subsystem4/1(Out5) -> Subsystem12/1(Ub), Subsystem2/1(Ub)
  Subsystem10/1(my2) -> my2/1, Subsystem4/1(In2)
  Subsystem6/1(mUp) -> Subsystem1/1(Qp), Subsystem14/1(Qp)
  Subsystem7/2(Out1) -> y1/1
  Subsystem7/3(Out2) -> vol1/1
  Subsystem10/2(yy2) -> y2/1
  Subsystem10/3(vol2) -> vol2/1

== system two_tank_simple/faultless3/FAULTLESS FAULT ==
  note: y2
  note: y1
  note: Ub
  note: Up
  note: Qvo
      | To users
  note: Qp
  note: Qvb
  Constant : Constant  Value=yo
  Subsystem1 : Subsystem
      mask Display: disp('TANK 1')
  Subsystem10 : Subsystem
      mask Display: disp('Sensor\n y2')
  Subsystem11 : Subsystem
      mask Display: disp('Controller 1')
  Subsystem12 : Subsystem
      mask Display: disp('Sensor\n Ub')
  Subsystem13 : Subsystem
      mask Display: disp('Sensor\n Up')
  Subsystem14 : Subsystem
      mask Display: disp('Sensor\n Qp')
  Subsystem2 : Subsystem
      mask Display: disp('Valve B')
  Subsystem3 : Subsystem
      mask Display: disp('Valve O')
  Subsystem4 : Subsystem
      mask Display: disp('Controller2')
  Subsystem6 : Subsystem
      mask Display: disp('Pump')
  Subsystem7 : Subsystem
      mask Display: disp('Sensor\n y1')
  Subsystem8 : Subsystem
      mask Display: disp('TANK 2')
  Subsystem9 : Subsystem
      mask Display: disp('OPERATOR\nSET')
  mQp : Outport
  mUb : Outport  Port=2
  "Uo " : Outport  Port=3
  my1 : Outport  Port=4
  my2 : Outport  Port=5
  h1c : Outport  Port=6
  mUp : Outport  Port=7
  mQ0 : Outport  Port=8
  y1 : Outport  Port=9
  vol1 : Outport  Port=10
  y2 : Outport  Port=11
  vol2 : Outport  Port=12
  wires:
  Subsystem1/1(y1) -> Subsystem2/2(y1), Subsystem7/1(In1)
  Subsystem12/1(mUb) -> mUb/1
  Subsystem3/1(Qv0) -> mQ0/1, Subsystem8/1(Qvo)
  Constant/1 -> Subsystem3/3(y0)
  Subsystem13/1(mUp) -> mUp/1
  Subsystem8/1(y2) -> Subsystem10/1(In1), Subsystem3/2(y2), Subsystem2/3(y2)
  Subsystem2/1(QVb) -> Subsystem8/2(Qvb), Subsystem1/2(Qvb)
  Subsystem11/1(mUp) -> Subsystem13/1(Up), Subsystem6/1(Up)
  Subsystem9/1(Out3) -> Subsystem11/1(h1c), h1c/1
  Subsystem9/2(Out1) -> "Uo "/1, Subsystem3/1(U0)
  Subsystem7/1(Out5) -> Subsystem11/2(my1), my1/1
  Subsystem14/1(mQp) -> mQp/1
  Subsystem4/1(Out5) -> Subsystem12/1(Ub), Subsystem2/1(Ub)
  Subsystem10/1(Out5) -> my2/1, Subsystem4/1(In2)
  Subsystem6/1(mUp) -> Subsystem1/1(Qp), Subsystem14/1(Qp)
  Subsystem7/2(Out1) -> y1/1
  Subsystem7/3(Out2) -> vol1/1
  Subsystem10/2(Out1) -> y2/1
  Subsystem10/3(Out2) -> vol2/1

== system two_tank_simple/mUp fault/FAULTLESS FAULT ==
  note: y2
  note: y1
  note: Ub
  note: Up
  note: Qvo
      | To users
  note: Qp
  note: Qvb
  Constant : Constant  Value=yo
  Subsystem1 : Subsystem
      mask Display: disp('TANK 1')
  Subsystem10 : Subsystem
      mask Display: disp('Sensor\n y2')
  Subsystem11 : Subsystem
      mask Display: disp('Controller 1')
  Subsystem12 : Subsystem
      mask Display: disp('Sensor\n Ub')
  Subsystem13 : Subsystem
      mask Display: disp('Sensor\n Up')
  Subsystem14 : Subsystem
      mask Display: disp('Sensor\n Qp')
  Subsystem2 : Subsystem
      mask Display: disp('Valve B')
  Subsystem3 : Subsystem
      mask Display: disp('Valve O')
  Subsystem4 : Subsystem
      mask Display: disp('Controller2')
  Subsystem6 : Subsystem
      mask Display: disp('Pump')
  Subsystem7 : Subsystem
      mask Display: disp('Sensor\n y1')
  Subsystem8 : Subsystem
      mask Display: disp('TANK 2')
  Subsystem9 : Subsystem
      mask Display: disp('OPERATOR\nSET')
  mQp : Outport
  mUb : Outport  Port=2
  "Uo " : Outport  Port=3
  my1 : Outport  Port=4
  my2 : Outport  Port=5
  h1c : Outport  Port=6
  mUp : Outport  Port=7
  mQ0 : Outport  Port=8
  vol1 : Outport  Port=9
  y1 : Outport  Port=10
  y2 : Outport  Port=11
  vol2 : Outport  Port=12
  wires:
  Subsystem1/1(y1) -> Subsystem2/2(y1), Subsystem7/1(In1)
  Subsystem12/1(mUb) -> mUb/1
  Subsystem3/1(Qv0) -> mQ0/1, Subsystem8/1(Qvo)
  Constant/1 -> Subsystem3/3(y0)
  Subsystem13/1(mUp) -> mUp/1
  Subsystem8/1(y2) -> Subsystem3/2(y2), Subsystem2/3(y2), Subsystem10/1(y2)
  Subsystem2/1(QVb) -> Subsystem8/2(Qvb), Subsystem1/2(Qvb)
  Subsystem11/1(mUp) -> Subsystem13/1(Up), Subsystem6/1(Up)
  Subsystem9/1(Out3) -> Subsystem11/1(h1c), h1c/1
  Subsystem9/2(Out1) -> "Uo "/1, Subsystem3/1(U0)
  Subsystem7/1(Out5) -> Subsystem11/2(my1), my1/1
  Subsystem14/1(mQp) -> mQp/1
  Subsystem4/1(Out5) -> Subsystem12/1(Ub), Subsystem2/1(Ub)
  Subsystem10/1(my2) -> my2/1, Subsystem4/1(In2)
  Subsystem6/1(mUp) -> Subsystem1/1(Qp), Subsystem14/1(Qp)
  Subsystem7/3(Out2) -> y1/1
  Subsystem7/2(Out1) -> vol1/1
  Subsystem10/3(vol2) -> vol2/1
  Subsystem10/2(yy2) -> y2/1

== system two_tank_simple/my1 fault/FAULTLESS FAULT ==
  note: y2
  note: y1
  note: Ub
  note: Up
  note: Qvo
      | To users
  note: Qp
  note: Qvb
  Constant : Constant  Value=yo
  Subsystem1 : Subsystem
      mask Display: disp('TANK 1')
  Subsystem10 : Subsystem
      mask Display: disp('Sensor\n y2')
  Subsystem11 : Subsystem
      mask Display: disp('Controller 1')
  Subsystem12 : Subsystem
      mask Display: disp('Sensor\n Ub')
  Subsystem13 : Subsystem
      mask Display: disp('Sensor\n Up')
  Subsystem14 : Subsystem
      mask Display: disp('Sensor\n Qp')
  Subsystem2 : Subsystem
      mask Display: disp('Valve B')
  Subsystem3 : Subsystem
      mask Display: disp('Valve O')
  Subsystem4 : Subsystem
      mask Display: disp('Controller2')
  Subsystem6 : Subsystem
      mask Display: disp('Pump')
  Subsystem7 : Subsystem
      mask Display: disp('Sensor\n y1')
  Subsystem8 : Subsystem
      mask Display: disp('TANK 2')
  Subsystem9 : Subsystem
      mask Display: disp('OPERATOR\nSET')
  mQp : Outport
  mUb : Outport  Port=2
  "Uo " : Outport  Port=3
  my1 : Outport  Port=4
  my2 : Outport  Port=5
  h1c : Outport  Port=6
  mUp : Outport  Port=7
  mq0 : Outport  Port=8
  y1 : Outport  Port=9
  vol1 : Outport  Port=10
  y2 : Outport  Port=11
  vol2 : Outport  Port=12
  wires:
  Subsystem1/1(y1) -> Subsystem2/2(y1), Subsystem7/1(In1)
  Subsystem12/1(mUb) -> mUb/1
  Subsystem3/1(Qv0) -> mq0/1, Subsystem8/1(Qvo)
  Constant/1 -> Subsystem3/3(y0)
  Subsystem13/1(mUp) -> mUp/1
  Subsystem8/1(y2) -> Subsystem3/2(y2), Subsystem2/3(y2), Subsystem10/1(y2)
  Subsystem2/1(QVb) -> Subsystem8/2(Qvb), Subsystem1/2(Qvb)
  Subsystem11/1(mUp) -> Subsystem13/1(Up), Subsystem6/1(Up)
  Subsystem9/1(Out3) -> Subsystem11/1(h1c), h1c/1
  Subsystem9/2(Out1) -> "Uo "/1, Subsystem3/1(U0)
  Subsystem7/1(Out5) -> Subsystem11/2(my1), my1/1
  Subsystem14/1(mQp) -> mQp/1
  Subsystem4/1(Out5) -> Subsystem12/1(Ub), Subsystem2/1(Ub)
  Subsystem10/1(my2) -> my2/1, Subsystem4/1(In2)
  Subsystem6/1(mUp) -> Subsystem1/1(Qp), Subsystem14/1(Qp)
  Subsystem7/2(Out1) -> y1/1
  Subsystem7/3(Out2) -> vol1/1
  Subsystem10/2(yy2) -> y2/1
  Subsystem10/3(vol2) -> vol2/1

== system two_tank_simple/my2 fault/FAULTLESS FAULT ==
  note: y2
  note: y1
  note: Ub
  note: Up
  note: Qvo
      | To users
  note: Qp
  note: Qvb
  Constant : Constant  Value=yo
  Subsystem1 : Subsystem
      mask Display: disp('TANK 1')
  Subsystem10 : Subsystem
      mask Display: disp('Sensor\n y2')
  Subsystem11 : Subsystem
      mask Display: disp('Controller 1')
  Subsystem12 : Subsystem
      mask Display: disp('Sensor\n Ub')
  Subsystem13 : Subsystem
      mask Display: disp('Sensor\n Up')
  Subsystem14 : Subsystem
      mask Display: disp('Sensor\n Qp')
  Subsystem2 : Subsystem
      mask Display: disp('Valve B')
  Subsystem3 : Subsystem
      mask Display: disp('Valve O')
  Subsystem4 : Subsystem
      mask Display: disp('Controller2')
  Subsystem6 : Subsystem
      mask Display: disp('Pump')
  Subsystem7 : Subsystem
      mask Display: disp('Sensor\n y1')
  Subsystem8 : Subsystem
      mask Display: disp('TANK 2')
  Subsystem9 : Subsystem
      mask Display: disp('OPERATOR\nSET')
  mQp : Outport
  mUb : Outport  Port=2
  "Uo " : Outport  Port=3
  my1 : Outport  Port=4
  my2 : Outport  Port=5
  h1c : Outport  Port=6
  mUp : Outport  Port=7
  mq0 : Outport  Port=8
  y1 : Outport  Port=9
  vol1 : Outport  Port=10
  y2 : Outport  Port=11
  vol2 : Outport  Port=12
  wires:
  Subsystem1/1(y1) -> Subsystem2/2(y1), Subsystem7/1(In1)
  Subsystem12/1(mUb) -> mUb/1
  Subsystem3/1(Qv0) -> mq0/1, Subsystem8/1(Qvo)
  Constant/1 -> Subsystem3/3(y0)
  Subsystem13/1(mUp) -> mUp/1
  Subsystem8/1(y2) -> Subsystem3/2(y2), Subsystem2/3(y2), Subsystem10/1(y2)
  Subsystem2/1(QVb) -> Subsystem8/2(Qvb), Subsystem1/2(Qvb)
  Subsystem11/1(mUp) -> Subsystem13/1(Up), Subsystem6/1(Up)
  Subsystem9/1(Out3) -> Subsystem11/1(h1c), h1c/1
  Subsystem9/2(Out1) -> "Uo "/1, Subsystem3/1(U0)
  Subsystem7/1(Out5) -> Subsystem11/2(my1), my1/1
  Subsystem14/1(mQp) -> mQp/1
  Subsystem4/1(Out5) -> Subsystem12/1(Ub), Subsystem2/1(Ub)
  Subsystem10/1(my2) -> my2/1, Subsystem4/1(In2)
  Subsystem6/1(mUp) -> Subsystem1/1(Qp), Subsystem14/1(Qp)
  Subsystem7/2(Out1) -> y1/1
  Subsystem7/3(Out2) -> vol1/1
  Subsystem10/2(yy2) -> y2/1
  Subsystem10/3(vol2) -> vol2/1

== system two_tank_simple/pump fault/FAULTLESS FAULT ==
  note: y2
  note: y1
  note: Ub
  note: Up
  note: Qvo
      | To users
  note: Qp
  note: Qvb
  Constant : Constant  Value=yo
  Subsystem1 : Subsystem
      mask Display: disp('TANK 1')
  Subsystem10 : Subsystem
      mask Display: disp('Sensor\n y2')
  Subsystem11 : Subsystem
      mask Display: disp('Controller 1')
  Subsystem12 : Subsystem
      mask Display: disp('Sensor\n Ub')
  Subsystem13 : Subsystem
      mask Display: disp('Sensor\n Up')
  Subsystem14 : Subsystem
      mask Display: disp('Sensor\n Qp')
  Subsystem2 : Subsystem
      mask Display: disp('Valve B')
  Subsystem3 : Subsystem
      mask Display: disp('Valve O')
  Subsystem4 : Subsystem
      mask Display: disp('Controller2')
  Subsystem6 : Subsystem
      mask Display: disp('Pump')
  Subsystem7 : Subsystem
      mask Display: disp('Sensor\n y1')
  Subsystem8 : Subsystem
      mask Display: disp('TANK 2')
  Subsystem9 : Subsystem
      mask Display: disp('OPERATOR\nSET')
  mQp : Outport
  mUb : Outport  Port=2
  "Uo " : Outport  Port=3
  my1 : Outport  Port=4
  my2 : Outport  Port=5
  h1c : Outport  Port=6
  mUp : Outport  Port=7
  mq0 : Outport  Port=8
  y1 : Outport  Port=9
  vol1 : Outport  Port=10
  y2 : Outport  Port=11
  vol2 : Outport  Port=12
  wires:
  Subsystem1/1(y1) -> Subsystem2/2(y1), Subsystem7/1(In1)
  Subsystem12/1(mUb) -> mUb/1
  Subsystem3/1(Qv0) -> mq0/1, Subsystem8/1(Qvo)
  Constant/1 -> Subsystem3/3(y0)
  Subsystem13/1(mUp) -> mUp/1
  Subsystem8/1(y2) -> Subsystem3/2(y2), Subsystem2/3(y2), Subsystem10/1(y2)
  Subsystem2/1(QVb) -> Subsystem8/2(Qvb), Subsystem1/2(Qvb)
  Subsystem11/1(mUp) -> Subsystem13/1(Up), Subsystem6/1(Up)
  Subsystem9/1(Out3) -> Subsystem11/1(h1c), h1c/1
  Subsystem9/2(Out1) -> "Uo "/1, Subsystem3/1(U0)
  Subsystem7/1(Out5) -> Subsystem11/2(my1), my1/1
  Subsystem14/1(mQp) -> mQp/1
  Subsystem4/1(Out5) -> Subsystem12/1(Ub), Subsystem2/1(Ub)
  Subsystem10/1(my2) -> my2/1, Subsystem4/1(In2)
  Subsystem6/1(mUp) -> Subsystem1/1(Qp), Subsystem14/1(Qp)
  Subsystem10/3(vol2) -> vol2/1
  Subsystem10/2(yy2) -> y2/1
  Subsystem7/2(Out1) -> y1/1
  Subsystem7/3(Out2) -> vol1/1

== system two_tank_simple/T1 fault/FAULTLESS FAULT/Subsystem1 ==
  note: TANK T1 SIMULATION
  note: Qf1
  note: Faultless mode
  note: Faulty mode
      | water leak
  Qp : Inport
  Qvb : Inport  Port=2
  Clock2 : Clock
  Constant : Constant  Value=0
  Constant2 : Constant  Value=0
  Gain : Gain  Gain=1/A1  SaturateOnIntegerOverflow=on  OutDataTypeStr=Inherit: Same as input  ParamDataTypeStr=Inherit: Same as input
  Integrator2 : Integrator  InitialCondition=h1c_0
  Saturation1 : Saturate  UpperLimit=h1max  LowerLimit=0  LinearizeAsGain=off
  Selector : ManualSwitch  CurrentSetting=0
  Sum2 : Sum  Inputs=+--  InputSameDT=on  SaturateOnIntegerOverflow=on  OutDataTypeStr=Inherit: Same as first input
  Switch1 : Switch  Threshold=120
  Switch4 : Switch  Threshold=40
  flow leak : Constant  Value=Qf1
  y1 : Outport  InitialOutput=0
  wires:
  Gain/1 -> Integrator2/1
  Sum2/1 -> Gain/1
  Qp/1 -> Sum2/1
  Qvb/1 -> Sum2/2
  Clock2/1 -> Switch4/2, Switch1/2
  flow leak/1 -> Switch4/1
  Constant/1 -> Switch4/3, Switch1/1
  Switch4/1 -> Switch1/3
  Selector/1 -> Sum2/3
  Switch1/1 -> Selector/1
  Constant2/1 -> Selector/2
  Integrator2/1 -> Saturation1/1
  Saturation1/1 -> y1/1

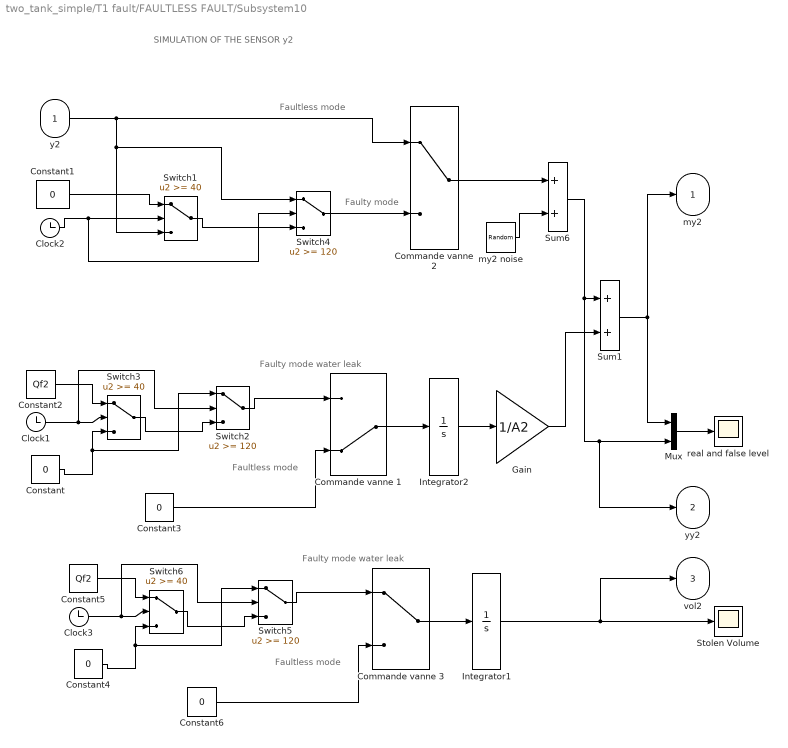
== system two_tank_simple/T1 fault/FAULTLESS FAULT/Subsystem10 ==
  note: SIMULATION OF THE SENSOR y2
  note: Faultless mode
  note: Faulty mode
  note: Faultless mode
  note: Faulty mode
      | water leak
  note: Faultless mode
  note: Faulty mode
      | water leak
  y2 : Inport
  Clock1 : Clock
  Clock2 : Clock
  Clock3 : Clock
  Commande vanne 1 : ManualSwitch  CurrentSetting=0
  Commande vanne 2 : ManualSwitch
  Commande vanne 3 : ManualSwitch
  Constant{,1,3..4,6} (5 alike) : Constant  Value=0
  Constant2 : Constant  Value=Qf2
  Constant5 : Constant  Value=Qf2
  Gain : Gain  Gain=1/A2  SaturateOnIntegerOverflow=on  OutDataTypeStr=Inherit: Same as input  ParamDataTypeStr=Inherit: Same as input
  Integrator1 : Integrator
  Integrator2 : Integrator
  Mux : Mux  Inputs=2
  Stolen Volume : Scope
  Sum1 : Sum  InputSameDT=on  SaturateOnIntegerOverflow=on  OutDataTypeStr=Inherit: Same as first input
  Sum6 : Sum  InputSameDT=on  SaturateOnIntegerOverflow=on  OutDataTypeStr=Inherit: Same as first input
  Switch1 : Switch  Threshold=40
  Switch2 : Switch  Threshold=120
  Switch3 : Switch  Threshold=40
  Switch4 : Switch  Threshold=120
  Switch5 : Switch  Threshold=120
  Switch6 : Switch  Threshold=40
  my2 noise : UniformRandomNumber  Minimum=-rate_noise_my2  Maximum=rate_noise_my2  SampleTime=0
  "real and false level " : Scope
  my2 : Outport  InitialOutput=0
  yy2 : Outport  Port=2  InitialOutput=0
  vol2 : Outport  Port=3  InitialOutput=0
  wires:
  my2 noise/1 -> Sum6/2
  Commande vanne 2/1 -> Sum6/1
  y2/1 -> Commande vanne 2/1, Switch1/3, Switch4/1
  Switch4/1 -> Commande vanne 2/2
  Switch1/1 -> Switch4/3
  Constant1/1 -> Switch1/1
  Clock2/1 -> Switch4/2, Switch1/2
  Clock1/1 -> Switch3/2, Switch2/2
  Constant2/1 -> Switch3/1
  Constant/1 -> Switch3/3, Switch2/1
  Switch3/1 -> Switch2/3
  Switch2/1 -> Commande vanne 1/1
  Constant3/1 -> Commande vanne 1/2
  Sum6/1 -> yy2/1, Mux/2, Sum1/1
  Sum1/1 -> Mux/1, my2/1
  Integrator2/1 -> Gain/1
  Mux/1 -> "real and false level "/1
  Commande vanne 1/1 -> Integrator2/1
  Gain/1 -> Sum1/2
  Clock3/1 -> Switch6/2, Switch5/2
  Constant5/1 -> Switch6/1
  Constant4/1 -> Switch6/3, Switch5/1
  Switch6/1 -> Switch5/3
  Switch5/1 -> Commande vanne 3/1
  Constant6/1 -> Commande vanne 3/2
  Integrator1/1 -> vol2/1, Stolen Volume/1
  Commande vanne 3/1 -> Integrator1/1

== system two_tank_simple/T1 fault/FAULTLESS FAULT/Subsystem11 ==
  note: Faultless mode
  note: Faulty mode
  note: Up
  note: SIMULATION OF THE DIGITAL PI CONTROLLER
  h1c : Inport
  my1 : Inport  Port=2
  Clock2 : Clock
  Commande vanne 2 : ManualSwitch
  Constant1 : Constant  Value=0
  Digital PIController : DiscreteTransferFcn  Numerator=[(Ki*Te+Kp) -Kp]  Denominator=[1 -1]  SampleTime=Te
  Sum : Sum  Inputs=+-  InputSameDT=on  SaturateOnIntegerOverflow=on  OutDataTypeStr=Inherit: Same as first input
  Switch1 : Switch  Threshold=40
  Switch4 : Switch  Threshold=120
  Zero-Order Hold4 : ZeroOrderHold  SampleTime=Te
  mUp : Outport  InitialOutput=0
  wires:
  Switch4/1 -> Commande vanne 2/2
  Commande vanne 2/1 -> mUp/1
  Digital PIController/1 -> Switch4/1, Switch1/3, Commande vanne 2/1
  Switch1/1 -> Switch4/3
  Constant1/1 -> Switch1/1
  Clock2/1 -> Switch4/2, Switch1/2
  h1c/1 -> Sum/1
  my1/1 -> Sum/2
  Zero-Order Hold4/1 -> Digital PIController/1
  Sum/1 -> Zero-Order Hold4/1

== system two_tank_simple/T1 fault/FAULTLESS FAULT/Subsystem12 ==
  note: SIMULATION OF THE SENSOR Ub
  note: Faultless mode
  note: Faulty mode
  Ub : Inport
  Clock2 : Clock
  Commande vanne 2 : ManualSwitch
  Constant1 : Constant  Value=0
  Switch1 : Switch  Threshold=40
  Switch4 : Switch  Threshold=120
  mUb : Outport  InitialOutput=0
  wires:
  Clock2/1 -> Switch1/2, Switch4/2
  Constant1/1 -> Switch1/1
  Switch1/1 -> Switch4/3
  Switch4/1 -> Commande vanne 2/2
  Ub/1 -> Commande vanne 2/1, Switch1/3, Switch4/1
  Commande vanne 2/1 -> mUb/1

== system two_tank_simple/T1 fault/FAULTLESS FAULT/Subsystem13 ==
  note: SIMULATION OF THE SENSOR Up
  note: Faultless mode
  note: Faulty mode
  Up : Inport
  Clock2 : Clock
  Commande vanne 2 : ManualSwitch
  Constant1 : Constant  Value=0
  Sum1 : Sum  InputSameDT=on  SaturateOnIntegerOverflow=on  OutDataTypeStr=Inherit: Same as first input
  Switch1 : Switch  Threshold=40
  Switch4 : Switch  Threshold=120
  mUp noise : UniformRandomNumber  Minimum=-rate_noise_mUp  Maximum=rate_noise_mUp  SampleTime=0
  mUp : Outport  InitialOutput=0
  wires:
  Up/1 -> Commande vanne 2/1, Switch1/3, Switch4/1
  Clock2/1 -> Switch1/2, Switch4/2
  Constant1/1 -> Switch1/1
  Switch1/1 -> Switch4/3
  Switch4/1 -> Commande vanne 2/2
  Sum1/1 -> mUp/1
  mUp noise/1 -> Sum1/2
  Commande vanne 2/1 -> Sum1/1

== system two_tank_simple/T1 fault/FAULTLESS FAULT/Subsystem14 ==
  note: SIMULATION OF THE SENSOR Qp
  note: Faultless mode
  note: Faulty mode
  Qp : Inport
  Clock2 : Clock
  Commande vanne 2 : ManualSwitch
  Constant1 : Constant  Value=0
  Sum6 : Sum  InputSameDT=on  SaturateOnIntegerOverflow=on  OutDataTypeStr=Inherit: Same as first input
  Switch1 : Switch  Threshold=40
  Switch4 : Switch  Threshold=120
  mQp noise : UniformRandomNumber  Minimum=-rate_noise_mQp  Maximum=rate_noise_mQp  SampleTime=0
  mQp : Outport  InitialOutput=0
  wires:
  Sum6/1 -> mQp/1
  Clock2/1 -> Switch1/2, Switch4/2
  Constant1/1 -> Switch1/1
  Switch1/1 -> Switch4/3
  Qp/1 -> Commande vanne 2/1, Switch1/3, Switch4/1
  Commande vanne 2/1 -> Sum6/1
  Switch4/1 -> Commande vanne 2/2
  mQp noise/1 -> Sum6/2

== system two_tank_simple/T1 fault/FAULTLESS FAULT/Subsystem2 ==
  note: SIMULATION OF VALVE Vb
  note: sign(y1-y2)
  note: Valve fault
      | Vb=0: Valve Vb blocked closed
      | Vb1=1: Valve Vb blocked opened
  note: Faultless mode
  note: Faulty mode
  Ub : Inport
  y1 : Inport  Port=2
  y2 : Inport  Port=3
  Abs : Abs
  Clock2 : Clock
  Commande vanne 1 : ManualSwitch
  Commande vanne 2 : ManualSwitch
  Gain : Gain  Gain=Cvb  SaturateOnIntegerOverflow=on  OutDataTypeStr=Inherit: Same as input  ParamDataTypeStr=Inherit: Same as input
  Math Function : Math  Operator=sqrt  SignedPower=on
  Product1 : Product  InputSameDT=on  SaturateOnIntegerOverflow=on  OutDataTypeStr=Inherit: Same as first input
  Product2 : Product  InputSameDT=on  SaturateOnIntegerOverflow=on  OutDataTypeStr=Inherit: Same as first input
  Sign(x1-x2) : Signum
  Sum : Sum  Inputs=+-  InputSameDT=on  SaturateOnIntegerOverflow=on  OutDataTypeStr=Inherit: Same as first input
  Switch1 : Switch  Threshold=150
  Switch4 : Switch  Threshold=40
  Vb : Constant  Value=0
  Vb1 : Constant
  QVb : Outport  InitialOutput=0
  wires:
  Gain/1 -> Product1/1
  Product1/1 -> QVb/1
  Product2/1 -> Gain/1
  y1/1 -> Sum/1
  Sign(x1-x2)/1 -> Product2/1
  Math Function/1 -> Product2/2
  Abs/1 -> Math Function/1
  Sum/1 -> Abs/1, Sign(x1-x2)/1
  y2/1 -> Sum/2
  Vb/1 -> Commande vanne 1/1
  Vb1/1 -> Commande vanne 1/2
  Clock2/1 -> Switch4/2, Switch1/2
  Ub/1 -> Commande vanne 2/1, Switch4/3, Switch1/1
  Commande vanne 1/1 -> Switch4/1
  Switch1/1 -> Commande vanne 2/2
  Switch4/1 -> Switch1/3
  Commande vanne 2/1 -> Product1/2
